simulink model "gap_generation_platoon_alternative"  (R2019a)
settings: Solver=VariableStepAuto  StartTime=0.0  StopTime=50  RelTol=1e-3
libraries: simulink x35, autolibshared x7, powerlib_meascontrol x3
(part 2 of 3)

== system gap_generation_platoon_alternative/p3 ==
  leaderStates : Inport
  virtualLeaderStates : Inport  Port=2
  lcFlag : Inport  Port=3
  activate ACC-v : Inport  Port=4
  ACC : Subsystem
  ACC-v : Subsystem
  AND : Logic  Inputs=3  IconShape=distinctive  AllPortsSameDT=off  OutDataTypeStr=boolean
  Abs : Abs
  Abs1 : Abs  ZeroCross=off
  Bus Creator : BusCreator  Inputs=4
  Bus Selector : BusSelector  OutputSignals=InertFrm.RearAxl.Disp.X,InertFrm.RearAxl.Disp.Y,InertFrm.RearAxl.Vel.Xdot
  Compare To Constant : simulink/Logic and Bit Operations/Compare To Constant  relop=<=  const=0.5  OutDataTypeStr=boolean
  Compare To Constant1 : simulink/Logic and Bit Operations/Compare To Constant  relop=<=  const=0.5  OutDataTypeStr=boolean
  Constant : Constant  Value=0
  Constant1 : Constant  Value=maxAcceleration+1
  Constant2 : Constant  Value=0
  Gain : Gain  Gain=m/2
  Min : MinMax  Inputs=2
  Mux1 : Mux  Inputs=6
  On Delay : powerlib_meascontrol/Logic/On Delay  DelayType=On delay  delay=1  ic=0  Ts=0
      settings: SourceProductName=Simscape Electrical
  Scope : Scope  NumInputPorts=2
  Signal Specification : SignalSpecification  Dimensions=1
  Switch : Switch  Criteria=u2 > Threshold
  Terminator : Terminator
  Transport Delay : TransportDelay
  Triggered Subsystem : Subsystem  TreatAsAtomicUnit=on
  Vehicle Body 3DOF Single Track : autolibshared/Vehicle Body 3DOF Single Track  trackMode=Single (bicycle)  inputMode=External longitudinal forces  frontSteerMode=on  rearSteerMode=off  windMode=off  muMode=off  extFMode=off  extMMode=off  extXo=off  extpsio=off  extxdoto=off  extro=off  extYo=off  extTamb=off  extydoto=off  aMode=2  NF=2  NR=2  m=m  a=lf  b=lr  h=0.35  X_o=x0  xdot_o=vx0  CalphaMode=off  sigmaMode=on  d=0  w=[1.4,1.4]  Cy_f=12e3  Cy_r=11e3  sigma_f=.1  sigma_r=.1  alpha_f_brk=[-.1 .1]  Cy_f_data=[-9e3 9e3]  alpha_r_brk=[-.1 .1]  Cy_r_data=[-9e3 9e3]  Y_o=y0  ydot_o=0  Izz=4000  psi_o=0  r_o=0  Af=2  Cd=.3  Cl=.1  Cpm=.1  beta_w=[0:0.01:0.3]  Cs=[0:0.03:0.9]  Cym=[0:0.01:0.3]  Pabs=101325  Tair=273  g=9.81  mu=1  xdot_tol=.01  Fznom=5000  Fxtire_sat=7e4  Fytire_sat=7e4  longOff=0  latOff=0  vertOff=0  wrapAng=off
      settings: SourceProductName=Powertrain Blockset  SourceProductBaseCode=PW
  states : Outport
  errors : Outport  Port=2
  gap : Outport  Port=3
  virtualErrors : Outport  Port=4
  virtualGap : Outport  Port=5
  gapRequest : Outport  Port=6
  wires:
  Bus Selector/3 -> Bus Creator/3  "<Xdot>"
  Bus Selector/1 -> Bus Creator/1  "<X>"
  Min/1 -> Signal Specification/1  "u"
  ACC/1(u) -> Min/1  "acc"
  Gain/1 -> Vehicle Body 3DOF Single Track/3, Vehicle Body 3DOF Single Track/2
  Constant/1 -> Vehicle Body 3DOF Single Track/1
  Vehicle Body 3DOF Single Track/1 -> Bus Selector/1
  Vehicle Body 3DOF Single Track/4 -> Mux1/3
  Vehicle Body 3DOF Single Track/3 -> Mux1/2
  Vehicle Body 3DOF Single Track/2 -> Mux1/1
  Vehicle Body 3DOF Single Track/5 -> Mux1/4
  Vehicle Body 3DOF Single Track/6 -> Mux1/5
  Vehicle Body 3DOF Single Track/7 -> Mux1/6
  Mux1/1 -> Terminator/1
  ACC/3(gap) -> gap/1
  Bus Creator/1 -> ACC/1(currentStates), ACC-v/1(currentStates), states/1
  leaderStates/1 -> ACC/2(leaderStates)
  virtualLeaderStates/1 -> ACC-v/2(leaderStates)
  ACC/2(errors) -> errors/1
  Switch/1 -> Min/2  "acc-v"
  ACC-v/1(u) -> Switch/1
  ACC-v/2(errors) -> virtualErrors/1
  ACC-v/3(gap) -> virtualGap/1
  Bus Selector/2 -> Bus Creator/2  "<Y>"
  Signal Specification/1 -> Transport Delay/1, Abs1/1, Bus Creator/4, Gain/1
  activate ACC-v/1 -> ACC-v/3(activate), Switch/2
  Constant1/1 -> Switch/3
  AND/1 -> Triggered Subsystem/Trigger
  Compare To Constant1/1 -> Scope/1, AND/1
  On Delay/1 -> AND/3, Triggered Subsystem/1(In1)
  Triggered Subsystem/1(Out1) -> Scope/2
  Compare To Constant/1 -> AND/2
  Transport Delay/1 -> Abs/1
  Abs/1 -> Compare To Constant/1
  Abs1/1 -> Compare To Constant1/1
  lcFlag/1 -> ACC-v/4(lcFlag), gapRequest/1, On Delay/1
  Constant2/1 -> ACC/3(lcFlag)

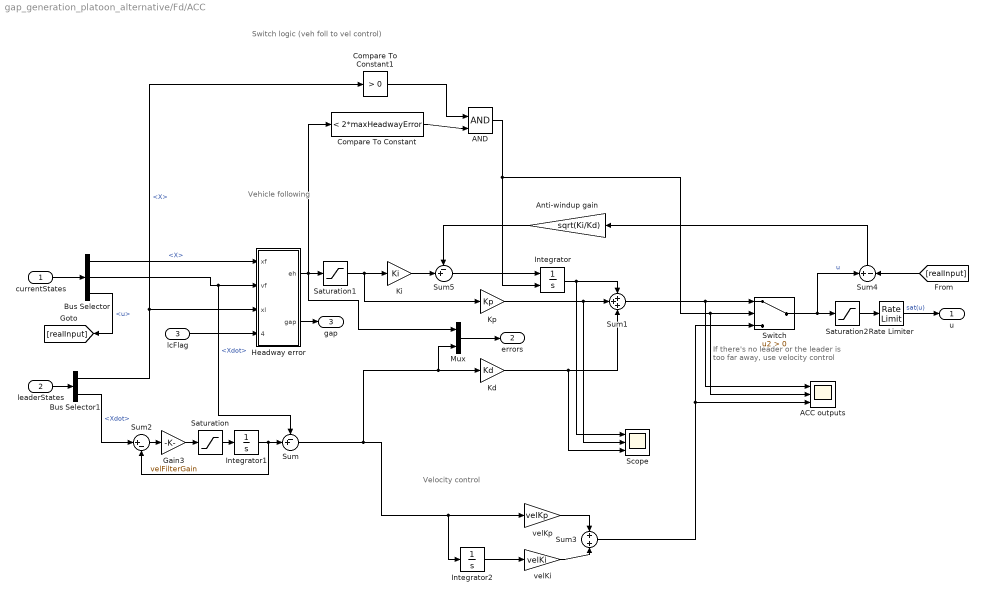
== system gap_generation_platoon_alternative/Fd/ACC ==
  note: Vehicle following
  note: Switch logic (veh foll to vel control)
  note: Velocity control
  note: If there's no leader or the leader
      | is too far away, use velocity control
  currentStates : Inport
  leaderStates : Inport  Port=2
  lcFlag : Inport  Port=3
  ACC outputs : Scope  NumInputPorts=3
  AND : Logic  IconShape=distinctive  AllPortsSameDT=off  OutDataTypeStr=boolean
  Anti-windup gain : Gain  Gain=sqrt(Ki/Kd)
  Bus Selector : BusSelector  OutputSignals=X,Xdot,u
  Bus Selector1 : BusSelector  OutputSignals=X,Xdot
  Compare To Constant : simulink/Logic and Bit Operations/Compare To Constant  relop=<  const=2*maxHeadwayError  OutDataTypeStr=boolean
  Compare To Constant1 : simulink/Logic and Bit Operations/Compare To Constant  relop=>  const=0  OutDataTypeStr=boolean
  Gain3 : Gain  Gain=velFilterGain
  Headway error : Subsystem
  Integrator : Integrator  ExternalReset=either
  Integrator1 : Integrator  InitialCondition=vx0
  Integrator2 : Integrator
  Kd : Gain  Gain=Kd
  Ki : Gain  Gain=Ki
  Kp : Gain  Gain=Kp
  Mux : Mux  Inputs=2
  Rate Limiter : RateLimiter  RisingSlewLimit=maxJerk  FallingSlewLimit=minJerk  SampleTimeMode=inherited
  Saturation : Saturate  UpperLimit=maxAcceleration  LowerLimit=minAcceleration
  Saturation1 : Saturate  UpperLimit=maxHeadwayError  LowerLimit=minHeadwayError
  Saturation2 : Saturate  UpperLimit=maxAcceleration  LowerLimit=minAcceleration
  Scope : Scope  NumInputPorts=3
  Sum : Sum  Inputs=-+|
  Sum1 : Sum  Inputs=+++
  Sum2 : Sum  Inputs=|+-
  Sum3 : Sum
  Sum4 : Sum  Inputs=+-
  Sum5 : Sum  Inputs=-+|
  Switch : Switch  Criteria=u2 > Threshold
  velKi : Gain  Gain=velKi
  velKp : Gain  Gain=velKp
  u : Outport
  errors : Outport  Port=2
  gap : Outport  Port=3
  wires:
  Headway error/1(eh) -> Mux/1, Compare To Constant/1, Saturation1/1
  Bus Selector/2 -> Headway error/2(vf), Sum/1  "<Xdot>"
  Kd/1 -> Scope/3, Sum1/3
  Kp/1 -> Scope/2, Sum1/2
  Gain3/1 -> Saturation/1
  Saturation/1 -> Integrator1/1
  Integrator1/1 -> Sum2/2, Sum/2
  Bus Selector1/2 -> Sum2/1  "<Xdot>"
  Sum2/1 -> Gain3/1
  Saturation1/1 -> Kp/1, Ki/1
  Headway error/2("gap ") -> gap/1
  Integrator2/1 -> velKi/1
  velKi/1 -> Sum3/2
  Switch/1 -> Sum4/1, Saturation2/1  "u"
  Sum1/1 -> Switch/1, ACC outputs/1
  Sum3/1 -> ACC outputs/3, Switch/3
  Sum/1 -> Mux/2, Kd/1, velKp/1, Integrator2/1
  Mux/1 -> errors/1
  Saturation2/1 -> Rate Limiter/1
  Sum4/1 -> Anti-windup gain/1
  Sum5/1 -> Integrator/1
  Rate Limiter/1 -> u/1  "sat(u)"
  velKp/1 -> Sum3/1
  Ki/1 -> Sum5/2
  Integrator/1 -> Sum1/1, Scope/1
  Anti-windup gain/1 -> Sum5/1
  AND/1 -> Integrator/2, Switch/2, ACC outputs/2
  Compare To Constant/1 -> AND/2
  Compare To Constant1/1 -> AND/1
  lcFlag/1 -> Headway error/4(lcFlag)
  currentStates/1 -> Bus Selector/1
  Bus Selector/1 -> Headway error/1(xf)  "<X>"
  leaderStates/1 -> Bus Selector1/1
  Bus Selector1/1 -> Compare To Constant1/1, Headway error/3(xl)  "<X>"
  Bus Selector/3 -> [realInput]  "<u>"
  [realInput] -> Sum4/2

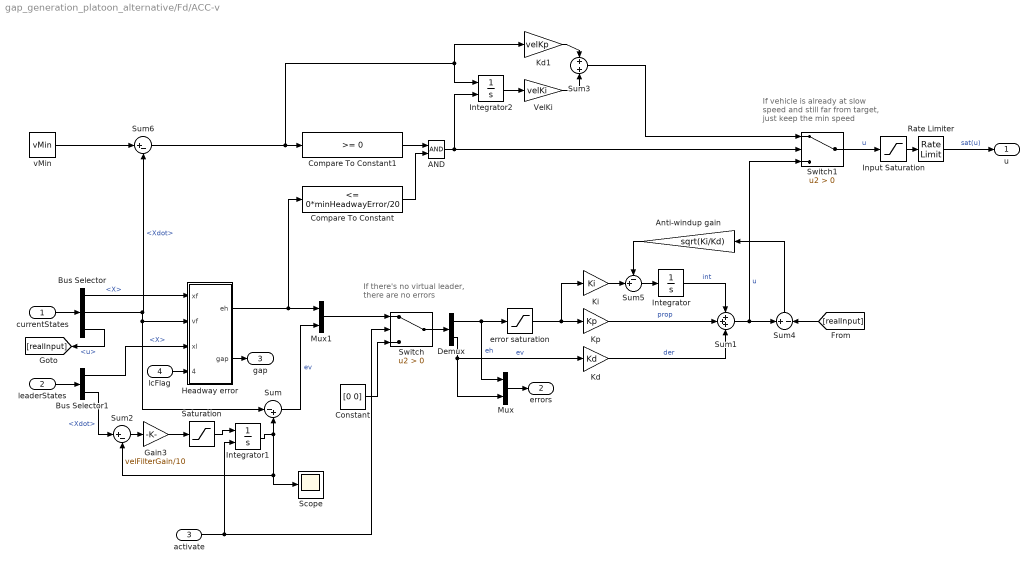
== system gap_generation_platoon_alternative/Fd/ACC-v ==
  note: If vehicle is already at slow
      | speed and still far from target,
      | just keep the min speed
  note: If there's no virtual leader,
      | there are no errors
  currentStates : Inport
  leaderStates : Inport  Port=2
  activate : Inport  Port=3
  lcFlag : Inport  Port=4
  AND : Logic  IconShape=distinctive  AllPortsSameDT=off  OutDataTypeStr=boolean
  Anti-windup gain : Gain  Gain=sqrt(Ki/Kd)
  Bus Selector : BusSelector  OutputSignals=X,Xdot,u
  Bus Selector1 : BusSelector  OutputSignals=X,Xdot
  Compare To Constant : simulink/Logic and Bit Operations/Compare To Constant  relop=<=  const=0*minHeadwayError/20  OutDataTypeStr=boolean
  Compare To Constant1 : simulink/Logic and Bit Operations/Compare To Constant  relop=>=  const=0  OutDataTypeStr=boolean
  Constant : Constant  Value=[0 0]
  Demux : Demux  Outputs=2
  Gain3 : Gain  Gain=velFilterGain/10
  Headway error : Subsystem
  Input Saturation : Saturate  UpperLimit=maxAcceleration/2  LowerLimit=minAcceleration/4
  Integrator : Integrator
  Integrator1 : Integrator  ExternalReset=rising  InitialCondition=vx0
  Integrator2 : Integrator  ExternalReset=rising
  Kd : Gain  Gain=Kd
  Kd1 : Gain  Gain=velKp
  Ki : Gain  Gain=Ki
  Kp : Gain  Gain=Kp
  Mux : Mux  Inputs=2
  Mux1 : Mux  Inputs=2
  Rate Limiter : RateLimiter  RisingSlewLimit=maxJerk/2  FallingSlewLimit=minJerk/3  SampleTimeMode=inherited
  Saturation : Saturate  UpperLimit=maxAcceleration  LowerLimit=minAcceleration
  Scope : Scope
  Sum : Sum  Inputs=|-+
  Sum1 : Sum  Inputs=+++
  Sum2 : Sum  Inputs=|+-
  Sum3 : Sum
  Sum4 : Sum  Inputs=+-
  Sum5 : Sum  Inputs=-+|
  Sum6 : Sum  Inputs=|+-
  Switch : Switch  Criteria=u2 > Threshold
  Switch1 : Switch  Criteria=u2 > Threshold
  VelKi : Gain  Gain=velKi
  error saturation : Saturate  UpperLimit=maxHeadwayError  LowerLimit=minHeadwayError/10
  vMin : Constant  Value=vMin
  u : Outport
  errors : Outport  Port=2
  gap : Outport  Port=3
  wires:
  Headway error/1(eh) -> Compare To Constant/1, Mux1/1
  Kd/1 -> Sum1/3  "der"
  Kp/1 -> Sum1/2  "prop"
  Gain3/1 -> Saturation/1
  Saturation/1 -> Integrator1/1
  Integrator1/1 -> Scope/1, Sum2/2, Sum/2
  Bus Selector1/2 -> Sum2/1  "<Xdot>"
  Sum2/1 -> Gain3/1
  Demux/1 -> Mux/1, error saturation/1  "eh"
  Headway error/2("gap ") -> gap/1
  Sum1/1 -> Switch1/3, Sum4/1  "u"
  Sum/1 -> Mux1/2  "ev"
  Mux/1 -> errors/1
  Input Saturation/1 -> Rate Limiter/1
  Integrator/1 -> Sum1/1  "int"
  Sum4/1 -> Anti-windup gain/1
  Ki/1 -> Sum5/2
  Anti-windup gain/1 -> Sum5/1
  Demux/2 -> Kd/1, Mux/2  "ev"
  Switch/1 -> Demux/1
  Mux1/1 -> Switch/1
  activate/1 -> Integrator1/2, Switch/2
  Constant/1 -> Switch/3
  Rate Limiter/1 -> u/1  "sat(u)"
  Compare To Constant1/1 -> AND/1
  Compare To Constant/1 -> AND/2
  Sum6/1 -> Integrator2/1, Kd1/1, Compare To Constant1/1
  Sum3/1 -> Switch1/1
  Integrator2/1 -> VelKi/1
  Kd1/1 -> Sum3/1
  VelKi/1 -> Sum3/2
  vMin/1 -> Sum6/1
  Switch1/1 -> Input Saturation/1  "u"
  error saturation/1 -> Kp/1, Ki/1
  Sum5/1 -> Integrator/1
  AND/1 -> Switch1/2, Integrator2/2
  [realInput] -> Sum4/2
  currentStates/1 -> Bus Selector/1
  Bus Selector/1 -> Headway error/1(xf)  "<X>"
  Bus Selector/2 -> Sum6/2, Headway error/2(vf), Sum/1  "<Xdot>"
  leaderStates/1 -> Bus Selector1/1
  Bus Selector1/1 -> Headway error/3(xl)  "<X>"
  Bus Selector/3 -> [realInput]  "<u>"
  lcFlag/1 -> Headway error/4(lcFlag)

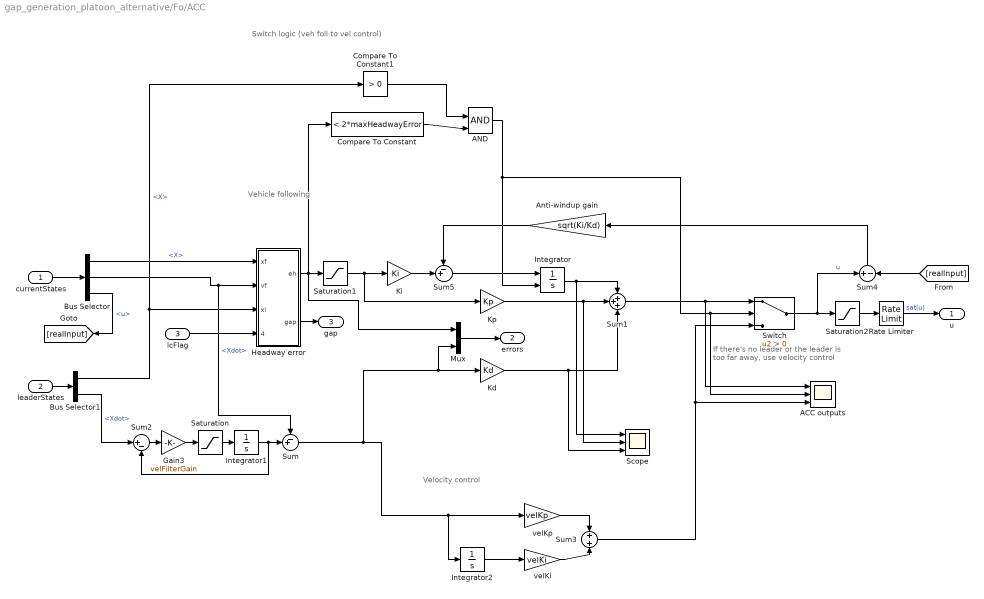
== system gap_generation_platoon_alternative/Fo/ACC ==
  note: Vehicle following
  note: Switch logic (veh foll to vel control)
  note: Velocity control
  note: If there's no leader or the leader
      | is too far away, use velocity control
  currentStates : Inport
  leaderStates : Inport  Port=2
  lcFlag : Inport  Port=3
  ACC outputs : Scope  NumInputPorts=3
  AND : Logic  IconShape=distinctive  AllPortsSameDT=off  OutDataTypeStr=boolean
  Anti-windup gain : Gain  Gain=sqrt(Ki/Kd)
  Bus Selector : BusSelector  OutputSignals=X,Xdot,u
  Bus Selector1 : BusSelector  OutputSignals=X,Xdot
  Compare To Constant : simulink/Logic and Bit Operations/Compare To Constant  relop=<  const=2*maxHeadwayError  OutDataTypeStr=boolean
  Compare To Constant1 : simulink/Logic and Bit Operations/Compare To Constant  relop=>  const=0  OutDataTypeStr=boolean
  Gain3 : Gain  Gain=velFilterGain
  Headway error : Subsystem
  Integrator : Integrator  ExternalReset=either
  Integrator1 : Integrator  InitialCondition=vx0
  Integrator2 : Integrator
  Kd : Gain  Gain=Kd
  Ki : Gain  Gain=Ki
  Kp : Gain  Gain=Kp
  Mux : Mux  Inputs=2
  Rate Limiter : RateLimiter  RisingSlewLimit=maxJerk  FallingSlewLimit=minJerk  SampleTimeMode=inherited
  Saturation : Saturate  UpperLimit=maxAcceleration  LowerLimit=minAcceleration
  Saturation1 : Saturate  UpperLimit=maxHeadwayError  LowerLimit=minHeadwayError
  Saturation2 : Saturate  UpperLimit=maxAcceleration  LowerLimit=minAcceleration
  Scope : Scope  NumInputPorts=3
  Sum : Sum  Inputs=-+|
  Sum1 : Sum  Inputs=+++
  Sum2 : Sum  Inputs=|+-
  Sum3 : Sum
  Sum4 : Sum  Inputs=+-
  Sum5 : Sum  Inputs=-+|
  Switch : Switch  Criteria=u2 > Threshold
  velKi : Gain  Gain=velKi
  velKp : Gain  Gain=velKp
  u : Outport
  errors : Outport  Port=2
  gap : Outport  Port=3
  wires:
  Headway error/1(eh) -> Mux/1, Compare To Constant/1, Saturation1/1
  Bus Selector/2 -> Headway error/2(vf), Sum/1  "<Xdot>"
  Kd/1 -> Scope/3, Sum1/3
  Kp/1 -> Scope/2, Sum1/2
  Gain3/1 -> Saturation/1
  Saturation/1 -> Integrator1/1
  Integrator1/1 -> Sum2/2, Sum/2
  Bus Selector1/2 -> Sum2/1  "<Xdot>"
  Sum2/1 -> Gain3/1
  Saturation1/1 -> Kp/1, Ki/1
  Headway error/2("gap ") -> gap/1
  Integrator2/1 -> velKi/1
  velKi/1 -> Sum3/2
  Switch/1 -> Sum4/1, Saturation2/1  "u"
  Sum1/1 -> Switch/1, ACC outputs/1
  Sum3/1 -> ACC outputs/3, Switch/3
  Sum/1 -> Mux/2, Kd/1, velKp/1, Integrator2/1
  Mux/1 -> errors/1
  Saturation2/1 -> Rate Limiter/1
  Sum4/1 -> Anti-windup gain/1
  Sum5/1 -> Integrator/1
  Rate Limiter/1 -> u/1  "sat(u)"
  velKp/1 -> Sum3/1
  Ki/1 -> Sum5/2
  Integrator/1 -> Sum1/1, Scope/1
  Anti-windup gain/1 -> Sum5/1
  AND/1 -> Integrator/2, Switch/2, ACC outputs/2
  Compare To Constant/1 -> AND/2
  Compare To Constant1/1 -> AND/1
  lcFlag/1 -> Headway error/4(lcFlag)
  currentStates/1 -> Bus Selector/1
  Bus Selector/1 -> Headway error/1(xf)  "<X>"
  leaderStates/1 -> Bus Selector1/1
  Bus Selector1/1 -> Compare To Constant1/1, Headway error/3(xl)  "<X>"
  Bus Selector/3 -> [realInput]  "<u>"
  [realInput] -> Sum4/2

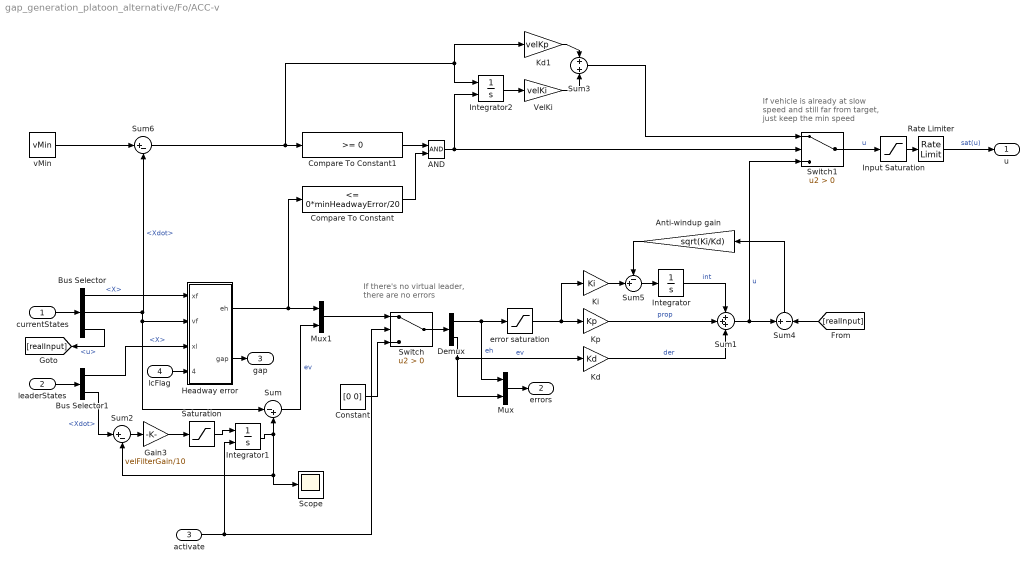
== system gap_generation_platoon_alternative/Fo/ACC-v ==
  note: If vehicle is already at slow
      | speed and still far from target,
      | just keep the min speed
  note: If there's no virtual leader,
      | there are no errors
  currentStates : Inport
  leaderStates : Inport  Port=2
  activate : Inport  Port=3
  lcFlag : Inport  Port=4
  AND : Logic  IconShape=distinctive  AllPortsSameDT=off  OutDataTypeStr=boolean
  Anti-windup gain : Gain  Gain=sqrt(Ki/Kd)
  Bus Selector : BusSelector  OutputSignals=X,Xdot,u
  Bus Selector1 : BusSelector  OutputSignals=X,Xdot
  Compare To Constant : simulink/Logic and Bit Operations/Compare To Constant  relop=<=  const=0*minHeadwayError/20  OutDataTypeStr=boolean
  Compare To Constant1 : simulink/Logic and Bit Operations/Compare To Constant  relop=>=  const=0  OutDataTypeStr=boolean
  Constant : Constant  Value=[0 0]
  Demux : Demux  Outputs=2
  Gain3 : Gain  Gain=velFilterGain/10
  Headway error : Subsystem
  Input Saturation : Saturate  UpperLimit=maxAcceleration/2  LowerLimit=minAcceleration/4
  Integrator : Integrator
  Integrator1 : Integrator  ExternalReset=rising  InitialCondition=vx0
  Integrator2 : Integrator  ExternalReset=rising
  Kd : Gain  Gain=Kd
  Kd1 : Gain  Gain=velKp
  Ki : Gain  Gain=Ki
  Kp : Gain  Gain=Kp
  Mux : Mux  Inputs=2
  Mux1 : Mux  Inputs=2
  Rate Limiter : RateLimiter  RisingSlewLimit=maxJerk/2  FallingSlewLimit=minJerk/3  SampleTimeMode=inherited
  Saturation : Saturate  UpperLimit=maxAcceleration  LowerLimit=minAcceleration
  Scope : Scope
  Sum : Sum  Inputs=|-+
  Sum1 : Sum  Inputs=+++
  Sum2 : Sum  Inputs=|+-
  Sum3 : Sum
  Sum4 : Sum  Inputs=+-
  Sum5 : Sum  Inputs=-+|
  Sum6 : Sum  Inputs=|+-
  Switch : Switch  Criteria=u2 > Threshold
  Switch1 : Switch  Criteria=u2 > Threshold
  VelKi : Gain  Gain=velKi
  error saturation : Saturate  UpperLimit=maxHeadwayError  LowerLimit=minHeadwayError/10
  vMin : Constant  Value=vMin
  u : Outport
  errors : Outport  Port=2
  gap : Outport  Port=3
  wires:
  Headway error/1(eh) -> Compare To Constant/1, Mux1/1
  Kd/1 -> Sum1/3  "der"
  Kp/1 -> Sum1/2  "prop"
  Gain3/1 -> Saturation/1
  Saturation/1 -> Integrator1/1
  Integrator1/1 -> Scope/1, Sum2/2, Sum/2
  Bus Selector1/2 -> Sum2/1  "<Xdot>"
  Sum2/1 -> Gain3/1
  Demux/1 -> Mux/1, error saturation/1  "eh"
  Headway error/2("gap ") -> gap/1
  Sum1/1 -> Switch1/3, Sum4/1  "u"
  Sum/1 -> Mux1/2  "ev"
  Mux/1 -> errors/1
  Input Saturation/1 -> Rate Limiter/1
  Integrator/1 -> Sum1/1  "int"
  Sum4/1 -> Anti-windup gain/1
  Ki/1 -> Sum5/2
  Anti-windup gain/1 -> Sum5/1
  Demux/2 -> Kd/1, Mux/2  "ev"
  Switch/1 -> Demux/1
  Mux1/1 -> Switch/1
  activate/1 -> Integrator1/2, Switch/2
  Constant/1 -> Switch/3
  Rate Limiter/1 -> u/1  "sat(u)"
  Compare To Constant1/1 -> AND/1
  Compare To Constant/1 -> AND/2
  Sum6/1 -> Integrator2/1, Kd1/1, Compare To Constant1/1
  Sum3/1 -> Switch1/1
  Integrator2/1 -> VelKi/1
  Kd1/1 -> Sum3/1
  VelKi/1 -> Sum3/2
  vMin/1 -> Sum6/1
  Switch1/1 -> Input Saturation/1  "u"
  error saturation/1 -> Kp/1, Ki/1
  Sum5/1 -> Integrator/1
  AND/1 -> Switch1/2, Integrator2/2
  [realInput] -> Sum4/2
  currentStates/1 -> Bus Selector/1
  Bus Selector/1 -> Headway error/1(xf)  "<X>"
  Bus Selector/2 -> Sum6/2, Headway error/2(vf), Sum/1  "<Xdot>"
  leaderStates/1 -> Bus Selector1/1
  Bus Selector1/1 -> Headway error/3(xl)  "<X>"
  Bus Selector/3 -> [realInput]  "<u>"
  lcFlag/1 -> Headway error/4(lcFlag)

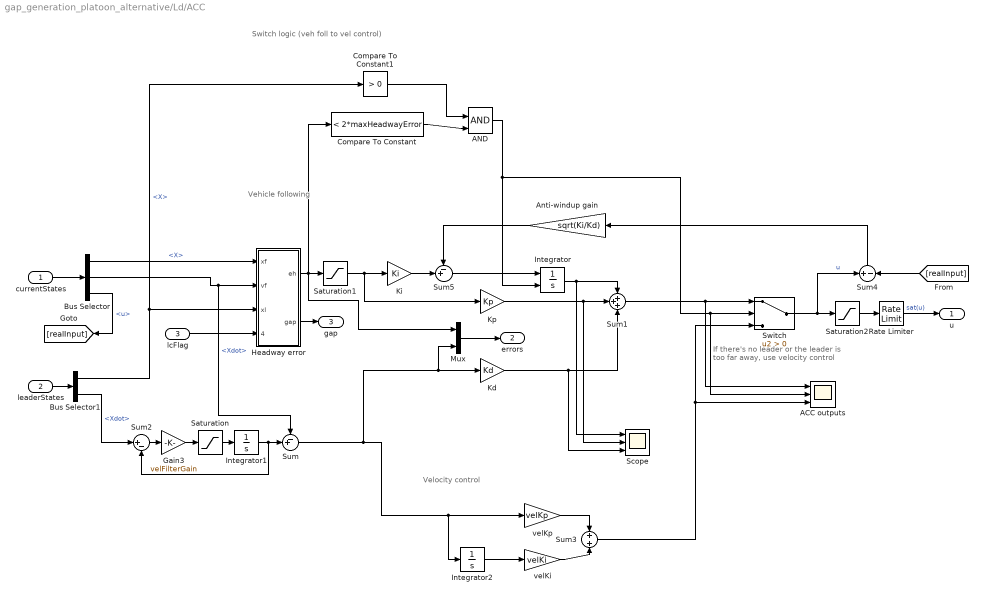
== system gap_generation_platoon_alternative/Ld/ACC ==
  note: Vehicle following
  note: Switch logic (veh foll to vel control)
  note: Velocity control
  note: If there's no leader or the leader
      | is too far away, use velocity control
  currentStates : Inport
  leaderStates : Inport  Port=2
  lcFlag : Inport  Port=3
  ACC outputs : Scope  NumInputPorts=3
  AND : Logic  IconShape=distinctive  AllPortsSameDT=off  OutDataTypeStr=boolean
  Anti-windup gain : Gain  Gain=sqrt(Ki/Kd)
  Bus Selector : BusSelector  OutputSignals=X,Xdot,u
  Bus Selector1 : BusSelector  OutputSignals=X,Xdot
  Compare To Constant : simulink/Logic and Bit Operations/Compare To Constant  relop=<  const=2*maxHeadwayError  OutDataTypeStr=boolean
  Compare To Constant1 : simulink/Logic and Bit Operations/Compare To Constant  relop=>  const=0  OutDataTypeStr=boolean
  Gain3 : Gain  Gain=velFilterGain
  Headway error : Subsystem
  Integrator : Integrator  ExternalReset=either
  Integrator1 : Integrator  InitialCondition=vx0
  Integrator2 : Integrator
  Kd : Gain  Gain=Kd
  Ki : Gain  Gain=Ki
  Kp : Gain  Gain=Kp
  Mux : Mux  Inputs=2
  Rate Limiter : RateLimiter  RisingSlewLimit=maxJerk  FallingSlewLimit=minJerk  SampleTimeMode=inherited
  Saturation : Saturate  UpperLimit=maxAcceleration  LowerLimit=minAcceleration
  Saturation1 : Saturate  UpperLimit=maxHeadwayError  LowerLimit=minHeadwayError
  Saturation2 : Saturate  UpperLimit=maxAcceleration  LowerLimit=minAcceleration
  Scope : Scope  NumInputPorts=3
  Sum : Sum  Inputs=-+|
  Sum1 : Sum  Inputs=+++
  Sum2 : Sum  Inputs=|+-
  Sum3 : Sum
  Sum4 : Sum  Inputs=+-
  Sum5 : Sum  Inputs=-+|
  Switch : Switch  Criteria=u2 > Threshold
  velKi : Gain  Gain=velKi
  velKp : Gain  Gain=velKp
  u : Outport
  errors : Outport  Port=2
  gap : Outport  Port=3
  wires:
  Headway error/1(eh) -> Mux/1, Compare To Constant/1, Saturation1/1
  Bus Selector/2 -> Headway error/2(vf), Sum/1  "<Xdot>"
  Kd/1 -> Scope/3, Sum1/3
  Kp/1 -> Scope/2, Sum1/2
  Gain3/1 -> Saturation/1
  Saturation/1 -> Integrator1/1
  Integrator1/1 -> Sum2/2, Sum/2
  Bus Selector1/2 -> Sum2/1  "<Xdot>"
  Sum2/1 -> Gain3/1
  Saturation1/1 -> Kp/1, Ki/1
  Headway error/2("gap ") -> gap/1
  Integrator2/1 -> velKi/1
  velKi/1 -> Sum3/2
  Switch/1 -> Sum4/1, Saturation2/1  "u"
  Sum1/1 -> Switch/1, ACC outputs/1
  Sum3/1 -> ACC outputs/3, Switch/3
  Sum/1 -> Mux/2, Kd/1, velKp/1, Integrator2/1
  Mux/1 -> errors/1
  Saturation2/1 -> Rate Limiter/1
  Sum4/1 -> Anti-windup gain/1
  Sum5/1 -> Integrator/1
  Rate Limiter/1 -> u/1  "sat(u)"
  velKp/1 -> Sum3/1
  Ki/1 -> Sum5/2
  Integrator/1 -> Sum1/1, Scope/1
  Anti-windup gain/1 -> Sum5/1
  AND/1 -> Integrator/2, Switch/2, ACC outputs/2
  Compare To Constant/1 -> AND/2
  Compare To Constant1/1 -> AND/1
  lcFlag/1 -> Headway error/4(lcFlag)
  currentStates/1 -> Bus Selector/1
  Bus Selector/1 -> Headway error/1(xf)  "<X>"
  leaderStates/1 -> Bus Selector1/1
  Bus Selector1/1 -> Compare To Constant1/1, Headway error/3(xl)  "<X>"
  Bus Selector/3 -> [realInput]  "<u>"
  [realInput] -> Sum4/2

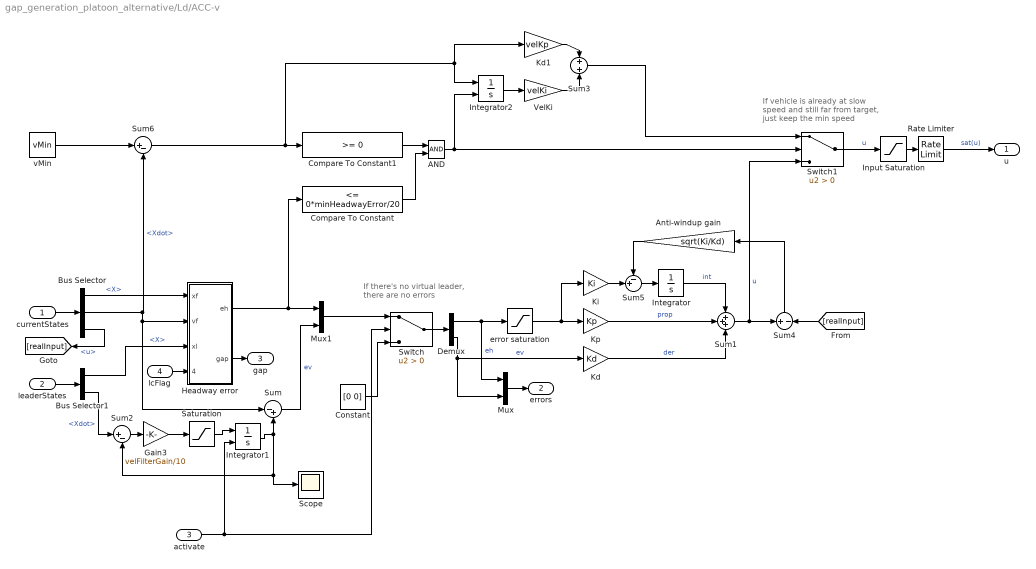
== system gap_generation_platoon_alternative/Ld/ACC-v ==
  note: If vehicle is already at slow
      | speed and still far from target,
      | just keep the min speed
  note: If there's no virtual leader,
      | there are no errors
  currentStates : Inport
  leaderStates : Inport  Port=2
  activate : Inport  Port=3
  lcFlag : Inport  Port=4
  AND : Logic  IconShape=distinctive  AllPortsSameDT=off  OutDataTypeStr=boolean
  Anti-windup gain : Gain  Gain=sqrt(Ki/Kd)
  Bus Selector : BusSelector  OutputSignals=X,Xdot,u
  Bus Selector1 : BusSelector  OutputSignals=X,Xdot
  Compare To Constant : simulink/Logic and Bit Operations/Compare To Constant  relop=<=  const=0*minHeadwayError/20  OutDataTypeStr=boolean
  Compare To Constant1 : simulink/Logic and Bit Operations/Compare To Constant  relop=>=  const=0  OutDataTypeStr=boolean
  Constant : Constant  Value=[0 0]
  Demux : Demux  Outputs=2
  Gain3 : Gain  Gain=velFilterGain/10
  Headway error : Subsystem
  Input Saturation : Saturate  UpperLimit=maxAcceleration/2  LowerLimit=minAcceleration/4
  Integrator : Integrator
  Integrator1 : Integrator  ExternalReset=rising  InitialCondition=vx0
  Integrator2 : Integrator  ExternalReset=rising
  Kd : Gain  Gain=Kd
  Kd1 : Gain  Gain=velKp
  Ki : Gain  Gain=Ki
  Kp : Gain  Gain=Kp
  Mux : Mux  Inputs=2
  Mux1 : Mux  Inputs=2
  Rate Limiter : RateLimiter  RisingSlewLimit=maxJerk/2  FallingSlewLimit=minJerk/3  SampleTimeMode=inherited
  Saturation : Saturate  UpperLimit=maxAcceleration  LowerLimit=minAcceleration
  Scope : Scope
  Sum : Sum  Inputs=|-+
  Sum1 : Sum  Inputs=+++
  Sum2 : Sum  Inputs=|+-
  Sum3 : Sum
  Sum4 : Sum  Inputs=+-
  Sum5 : Sum  Inputs=-+|
  Sum6 : Sum  Inputs=|+-
  Switch : Switch  Criteria=u2 > Threshold
  Switch1 : Switch  Criteria=u2 > Threshold
  VelKi : Gain  Gain=velKi
  error saturation : Saturate  UpperLimit=maxHeadwayError  LowerLimit=minHeadwayError/10
  vMin : Constant  Value=vMin
  u : Outport
  errors : Outport  Port=2
  gap : Outport  Port=3
  wires:
  Headway error/1(eh) -> Compare To Constant/1, Mux1/1
  Kd/1 -> Sum1/3  "der"
  Kp/1 -> Sum1/2  "prop"
  Gain3/1 -> Saturation/1
  Saturation/1 -> Integrator1/1
  Integrator1/1 -> Scope/1, Sum2/2, Sum/2
  Bus Selector1/2 -> Sum2/1  "<Xdot>"
  Sum2/1 -> Gain3/1
  Demux/1 -> Mux/1, error saturation/1  "eh"
  Headway error/2("gap ") -> gap/1
  Sum1/1 -> Switch1/3, Sum4/1  "u"
  Sum/1 -> Mux1/2  "ev"
  Mux/1 -> errors/1
  Input Saturation/1 -> Rate Limiter/1
  Integrator/1 -> Sum1/1  "int"
  Sum4/1 -> Anti-windup gain/1
  Ki/1 -> Sum5/2
  Anti-windup gain/1 -> Sum5/1
  Demux/2 -> Kd/1, Mux/2  "ev"
  Switch/1 -> Demux/1
  Mux1/1 -> Switch/1
  activate/1 -> Integrator1/2, Switch/2
  Constant/1 -> Switch/3
  Rate Limiter/1 -> u/1  "sat(u)"
  Compare To Constant1/1 -> AND/1
  Compare To Constant/1 -> AND/2
  Sum6/1 -> Integrator2/1, Kd1/1, Compare To Constant1/1
  Sum3/1 -> Switch1/1
  Integrator2/1 -> VelKi/1
  Kd1/1 -> Sum3/1
  VelKi/1 -> Sum3/2
  vMin/1 -> Sum6/1
  Switch1/1 -> Input Saturation/1  "u"
  error saturation/1 -> Kp/1, Ki/1
  Sum5/1 -> Integrator/1
  AND/1 -> Switch1/2, Integrator2/2
  [realInput] -> Sum4/2
  currentStates/1 -> Bus Selector/1
  Bus Selector/1 -> Headway error/1(xf)  "<X>"
  Bus Selector/2 -> Sum6/2, Headway error/2(vf), Sum/1  "<Xdot>"
  leaderStates/1 -> Bus Selector1/1
  Bus Selector1/1 -> Headway error/3(xl)  "<X>"
  Bus Selector/3 -> [realInput]  "<u>"
  lcFlag/1 -> Headway error/4(lcFlag)

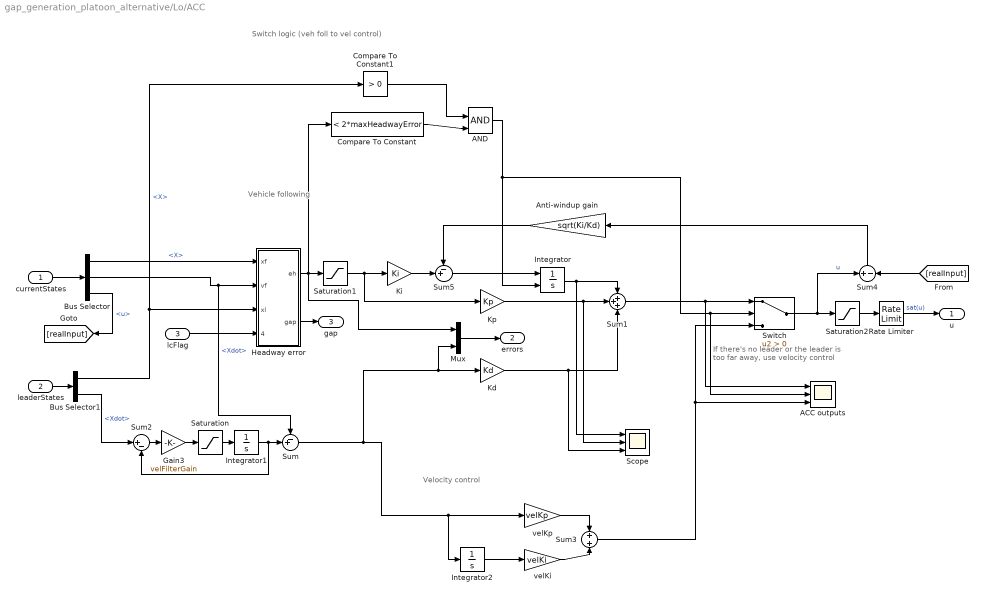
== system gap_generation_platoon_alternative/Lo/ACC ==
  note: Vehicle following
  note: Switch logic (veh foll to vel control)
  note: Velocity control
  note: If there's no leader or the leader
      | is too far away, use velocity control
  currentStates : Inport
  leaderStates : Inport  Port=2
  lcFlag : Inport  Port=3
  ACC outputs : Scope  NumInputPorts=3
  AND : Logic  IconShape=distinctive  AllPortsSameDT=off  OutDataTypeStr=boolean
  Anti-windup gain : Gain  Gain=sqrt(Ki/Kd)
  Bus Selector : BusSelector  OutputSignals=X,Xdot,u
  Bus Selector1 : BusSelector  OutputSignals=X,Xdot
  Compare To Constant : simulink/Logic and Bit Operations/Compare To Constant  relop=<  const=2*maxHeadwayError  OutDataTypeStr=boolean
  Compare To Constant1 : simulink/Logic and Bit Operations/Compare To Constant  relop=>  const=0  OutDataTypeStr=boolean
  Gain3 : Gain  Gain=velFilterGain
  Headway error : Subsystem
  Integrator : Integrator  ExternalReset=either
  Integrator1 : Integrator  InitialCondition=vx0
  Integrator2 : Integrator
  Kd : Gain  Gain=Kd
  Ki : Gain  Gain=Ki
  Kp : Gain  Gain=Kp
  Mux : Mux  Inputs=2
  Rate Limiter : RateLimiter  RisingSlewLimit=maxJerk  FallingSlewLimit=minJerk  SampleTimeMode=inherited
  Saturation : Saturate  UpperLimit=maxAcceleration  LowerLimit=minAcceleration
  Saturation1 : Saturate  UpperLimit=maxHeadwayError  LowerLimit=minHeadwayError
  Saturation2 : Saturate  UpperLimit=maxAcceleration  LowerLimit=minAcceleration
  Scope : Scope  NumInputPorts=3
  Sum : Sum  Inputs=-+|
  Sum1 : Sum  Inputs=+++
  Sum2 : Sum  Inputs=|+-
  Sum3 : Sum
  Sum4 : Sum  Inputs=+-
  Sum5 : Sum  Inputs=-+|
  Switch : Switch  Criteria=u2 > Threshold
  velKi : Gain  Gain=velKi
  velKp : Gain  Gain=velKp
  u : Outport
  errors : Outport  Port=2
  gap : Outport  Port=3
  wires:
  Headway error/1(eh) -> Mux/1, Compare To Constant/1, Saturation1/1
  Bus Selector/2 -> Headway error/2(vf), Sum/1  "<Xdot>"
  Kd/1 -> Scope/3, Sum1/3
  Kp/1 -> Scope/2, Sum1/2
  Gain3/1 -> Saturation/1
  Saturation/1 -> Integrator1/1
  Integrator1/1 -> Sum2/2, Sum/2
  Bus Selector1/2 -> Sum2/1  "<Xdot>"
  Sum2/1 -> Gain3/1
  Saturation1/1 -> Kp/1, Ki/1
  Headway error/2("gap ") -> gap/1
  Integrator2/1 -> velKi/1
  velKi/1 -> Sum3/2
  Switch/1 -> Sum4/1, Saturation2/1  "u"
  Sum1/1 -> Switch/1, ACC outputs/1
  Sum3/1 -> ACC outputs/3, Switch/3
  Sum/1 -> Mux/2, Kd/1, velKp/1, Integrator2/1
  Mux/1 -> errors/1
  Saturation2/1 -> Rate Limiter/1
  Sum4/1 -> Anti-windup gain/1
  Sum5/1 -> Integrator/1
  Rate Limiter/1 -> u/1  "sat(u)"
  velKp/1 -> Sum3/1
  Ki/1 -> Sum5/2
  Integrator/1 -> Sum1/1, Scope/1
  Anti-windup gain/1 -> Sum5/1
  AND/1 -> Integrator/2, Switch/2, ACC outputs/2
  Compare To Constant/1 -> AND/2
  Compare To Constant1/1 -> AND/1
  lcFlag/1 -> Headway error/4(lcFlag)
  currentStates/1 -> Bus Selector/1
  Bus Selector/1 -> Headway error/1(xf)  "<X>"
  leaderStates/1 -> Bus Selector1/1
  Bus Selector1/1 -> Compare To Constant1/1, Headway error/3(xl)  "<X>"
  Bus Selector/3 -> [realInput]  "<u>"
  [realInput] -> Sum4/2

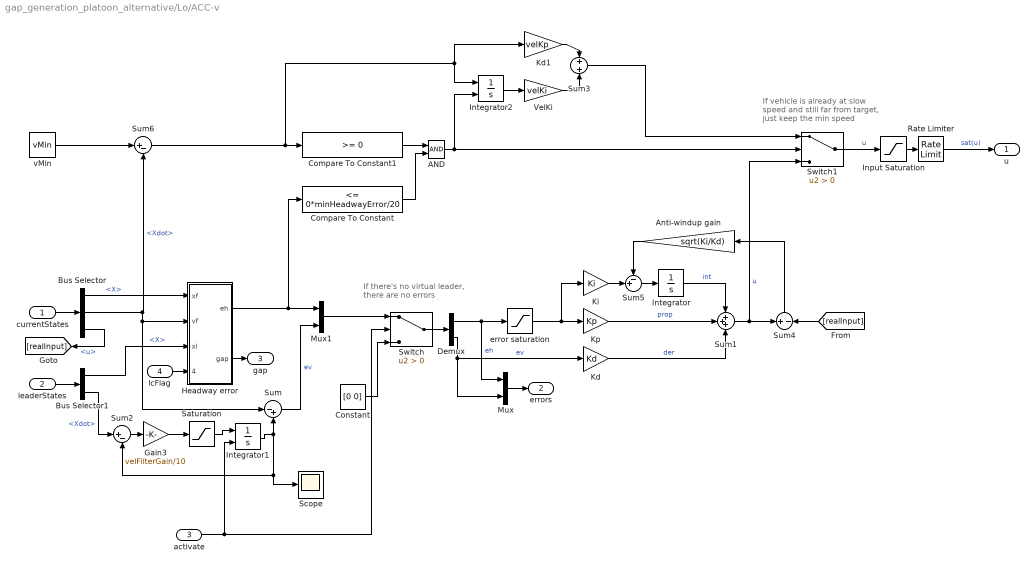
== system gap_generation_platoon_alternative/Lo/ACC-v ==
  note: If vehicle is already at slow
      | speed and still far from target,
      | just keep the min speed
  note: If there's no virtual leader,
      | there are no errors
  currentStates : Inport
  leaderStates : Inport  Port=2
  activate : Inport  Port=3
  lcFlag : Inport  Port=4
  AND : Logic  IconShape=distinctive  AllPortsSameDT=off  OutDataTypeStr=boolean
  Anti-windup gain : Gain  Gain=sqrt(Ki/Kd)
  Bus Selector : BusSelector  OutputSignals=X,Xdot,u
  Bus Selector1 : BusSelector  OutputSignals=X,Xdot
  Compare To Constant : simulink/Logic and Bit Operations/Compare To Constant  relop=<=  const=0*minHeadwayError/20  OutDataTypeStr=boolean
  Compare To Constant1 : simulink/Logic and Bit Operations/Compare To Constant  relop=>=  const=0  OutDataTypeStr=boolean
  Constant : Constant  Value=[0 0]
  Demux : Demux  Outputs=2
  Gain3 : Gain  Gain=velFilterGain/10
  Headway error : Subsystem
  Input Saturation : Saturate  UpperLimit=maxAcceleration/2  LowerLimit=minAcceleration/4
  Integrator : Integrator
  Integrator1 : Integrator  ExternalReset=rising  InitialCondition=vx0
  Integrator2 : Integrator  ExternalReset=rising
  Kd : Gain  Gain=Kd
  Kd1 : Gain  Gain=velKp
  Ki : Gain  Gain=Ki
  Kp : Gain  Gain=Kp
  Mux : Mux  Inputs=2
  Mux1 : Mux  Inputs=2
  Rate Limiter : RateLimiter  RisingSlewLimit=maxJerk/2  FallingSlewLimit=minJerk/3  SampleTimeMode=inherited
  Saturation : Saturate  UpperLimit=maxAcceleration  LowerLimit=minAcceleration
  Scope : Scope
  Sum : Sum  Inputs=|-+
  Sum1 : Sum  Inputs=+++
  Sum2 : Sum  Inputs=|+-
  Sum3 : Sum
  Sum4 : Sum  Inputs=+-
  Sum5 : Sum  Inputs=-+|
  Sum6 : Sum  Inputs=|+-
  Switch : Switch  Criteria=u2 > Threshold
  Switch1 : Switch  Criteria=u2 > Threshold
  VelKi : Gain  Gain=velKi
  error saturation : Saturate  UpperLimit=maxHeadwayError  LowerLimit=minHeadwayError/10
  vMin : Constant  Value=vMin
  u : Outport
  errors : Outport  Port=2
  gap : Outport  Port=3
  wires:
  Headway error/1(eh) -> Compare To Constant/1, Mux1/1
  Kd/1 -> Sum1/3  "der"
  Kp/1 -> Sum1/2  "prop"
  Gain3/1 -> Saturation/1
  Saturation/1 -> Integrator1/1
  Integrator1/1 -> Scope/1, Sum2/2, Sum/2
  Bus Selector1/2 -> Sum2/1  "<Xdot>"
  Sum2/1 -> Gain3/1
  Demux/1 -> Mux/1, error saturation/1  "eh"
  Headway error/2("gap ") -> gap/1
  Sum1/1 -> Switch1/3, Sum4/1  "u"
  Sum/1 -> Mux1/2  "ev"
  Mux/1 -> errors/1
  Input Saturation/1 -> Rate Limiter/1
  Integrator/1 -> Sum1/1  "int"
  Sum4/1 -> Anti-windup gain/1
  Ki/1 -> Sum5/2
  Anti-windup gain/1 -> Sum5/1
  Demux/2 -> Kd/1, Mux/2  "ev"
  Switch/1 -> Demux/1
  Mux1/1 -> Switch/1
  activate/1 -> Integrator1/2, Switch/2
  Constant/1 -> Switch/3
  Rate Limiter/1 -> u/1  "sat(u)"
  Compare To Constant1/1 -> AND/1
  Compare To Constant/1 -> AND/2
  Sum6/1 -> Integrator2/1, Kd1/1, Compare To Constant1/1
  Sum3/1 -> Switch1/1
  Integrator2/1 -> VelKi/1
  Kd1/1 -> Sum3/1
  VelKi/1 -> Sum3/2
  vMin/1 -> Sum6/1
  Switch1/1 -> Input Saturation/1  "u"
  error saturation/1 -> Kp/1, Ki/1
  Sum5/1 -> Integrator/1
  AND/1 -> Switch1/2, Integrator2/2
  [realInput] -> Sum4/2
  currentStates/1 -> Bus Selector/1
  Bus Selector/1 -> Headway error/1(xf)  "<X>"
  Bus Selector/2 -> Sum6/2, Headway error/2(vf), Sum/1  "<Xdot>"
  leaderStates/1 -> Bus Selector1/1
  Bus Selector1/1 -> Headway error/3(xl)  "<X>"
  Bus Selector/3 -> [realInput]  "<u>"
  lcFlag/1 -> Headway error/4(lcFlag)

== system gap_generation_platoon_alternative/p1/ACC ==
  note: Vehicle following
  note: Switch logic (veh foll to vel control)
  note: Velocity control
  note: If there's no leader or the leader
      | is too far away, use velocity control
  currentStates : Inport
  leaderStates : Inport  Port=2
  lcFlag : Inport  Port=3
  ACC outputs : Scope  NumInputPorts=3
  AND : Logic  IconShape=distinctive  AllPortsSameDT=off  OutDataTypeStr=boolean
  Anti-windup gain : Gain  Gain=sqrt(Ki/Kd)
  Bus Selector : BusSelector  OutputSignals=X,Xdot,u
  Bus Selector1 : BusSelector  OutputSignals=X,Xdot
  Compare To Constant : simulink/Logic and Bit Operations/Compare To Constant  relop=<  const=2*maxHeadwayError  OutDataTypeStr=boolean
  Compare To Constant1 : simulink/Logic and Bit Operations/Compare To Constant  relop=>  const=0  OutDataTypeStr=boolean
  Gain3 : Gain  Gain=velFilterGain
  Headway error : Subsystem
  Integrator : Integrator  ExternalReset=either
  Integrator1 : Integrator  InitialCondition=vx0
  Integrator2 : Integrator
  Kd : Gain  Gain=Kd
  Ki : Gain  Gain=Ki
  Kp : Gain  Gain=Kp
  Mux : Mux  Inputs=2
  Rate Limiter : RateLimiter  RisingSlewLimit=maxJerk  FallingSlewLimit=minJerk  SampleTimeMode=inherited
  Saturation : Saturate  UpperLimit=maxAcceleration  LowerLimit=minAcceleration
  Saturation1 : Saturate  UpperLimit=maxHeadwayError  LowerLimit=minHeadwayError
  Saturation2 : Saturate  UpperLimit=maxAcceleration  LowerLimit=minAcceleration
  Scope : Scope  NumInputPorts=3
  Sum : Sum  Inputs=-+|
  Sum1 : Sum  Inputs=+++
  Sum2 : Sum  Inputs=|+-
  Sum3 : Sum
  Sum4 : Sum  Inputs=+-
  Sum5 : Sum  Inputs=-+|
  Switch : Switch  Criteria=u2 > Threshold
  velKi : Gain  Gain=velKi
  velKp : Gain  Gain=velKp
  u : Outport
  errors : Outport  Port=2
  gap : Outport  Port=3
  wires:
  Headway error/1(eh) -> Mux/1, Compare To Constant/1, Saturation1/1
  Bus Selector/2 -> Headway error/2(vf), Sum/1  "<Xdot>"
  Kd/1 -> Scope/3, Sum1/3
  Kp/1 -> Scope/2, Sum1/2
  Gain3/1 -> Saturation/1
  Saturation/1 -> Integrator1/1
  Integrator1/1 -> Sum2/2, Sum/2
  Bus Selector1/2 -> Sum2/1  "<Xdot>"
  Sum2/1 -> Gain3/1
  Saturation1/1 -> Kp/1, Ki/1
  Headway error/2("gap ") -> gap/1
  Integrator2/1 -> velKi/1
  velKi/1 -> Sum3/2
  Switch/1 -> Sum4/1, Saturation2/1  "u"
  Sum1/1 -> Switch/1, ACC outputs/1
  Sum3/1 -> ACC outputs/3, Switch/3
  Sum/1 -> Mux/2, Kd/1, velKp/1, Integrator2/1
  Mux/1 -> errors/1
  Saturation2/1 -> Rate Limiter/1
  Sum4/1 -> Anti-windup gain/1
  Sum5/1 -> Integrator/1
  Rate Limiter/1 -> u/1  "sat(u)"
  velKp/1 -> Sum3/1
  Ki/1 -> Sum5/2
  Integrator/1 -> Sum1/1, Scope/1
  Anti-windup gain/1 -> Sum5/1
  AND/1 -> Integrator/2, Switch/2, ACC outputs/2
  Compare To Constant/1 -> AND/2
  Compare To Constant1/1 -> AND/1
  lcFlag/1 -> Headway error/4(lcFlag)
  currentStates/1 -> Bus Selector/1
  Bus Selector/1 -> Headway error/1(xf)  "<X>"
  leaderStates/1 -> Bus Selector1/1
  Bus Selector1/1 -> Compare To Constant1/1, Headway error/3(xl)  "<X>"
  Bus Selector/3 -> [realInput]  "<u>"
  [realInput] -> Sum4/2

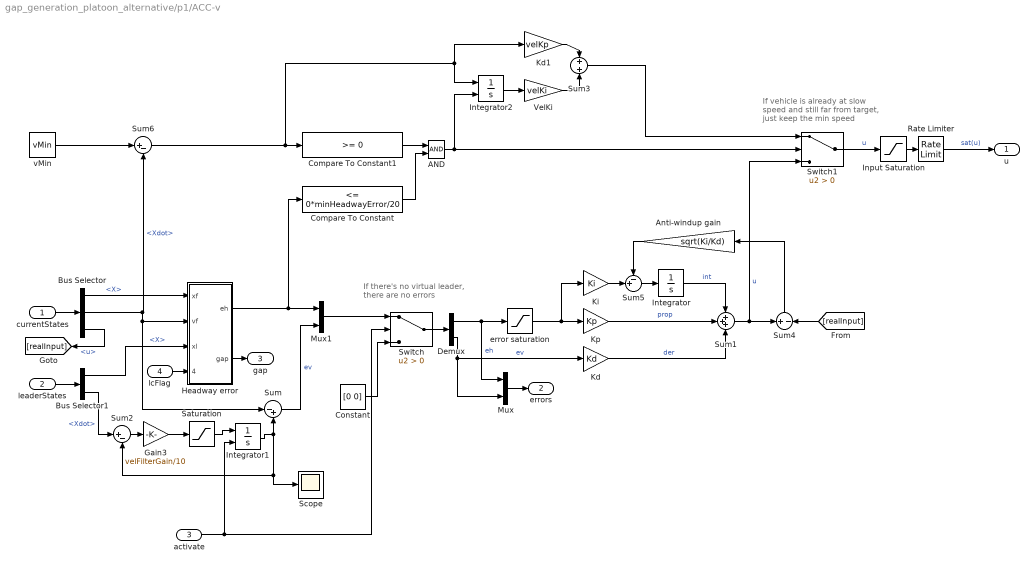
== system gap_generation_platoon_alternative/p1/ACC-v ==
  note: If vehicle is already at slow
      | speed and still far from target,
      | just keep the min speed
  note: If there's no virtual leader,
      | there are no errors
  currentStates : Inport
  leaderStates : Inport  Port=2
  activate : Inport  Port=3
  lcFlag : Inport  Port=4
  AND : Logic  IconShape=distinctive  AllPortsSameDT=off  OutDataTypeStr=boolean
  Anti-windup gain : Gain  Gain=sqrt(Ki/Kd)
  Bus Selector : BusSelector  OutputSignals=X,Xdot,u
  Bus Selector1 : BusSelector  OutputSignals=X,Xdot
  Compare To Constant : simulink/Logic and Bit Operations/Compare To Constant  relop=<=  const=0*minHeadwayError/20  OutDataTypeStr=boolean
  Compare To Constant1 : simulink/Logic and Bit Operations/Compare To Constant  relop=>=  const=0  OutDataTypeStr=boolean
  Constant : Constant  Value=[0 0]
  Demux : Demux  Outputs=2
  Gain3 : Gain  Gain=velFilterGain/10
  Headway error : Subsystem
  Input Saturation : Saturate  UpperLimit=maxAcceleration/2  LowerLimit=minAcceleration/4
  Integrator : Integrator
  Integrator1 : Integrator  ExternalReset=rising  InitialCondition=vx0
  Integrator2 : Integrator  ExternalReset=rising
  Kd : Gain  Gain=Kd
  Kd1 : Gain  Gain=velKp
  Ki : Gain  Gain=Ki
  Kp : Gain  Gain=Kp
  Mux : Mux  Inputs=2
  Mux1 : Mux  Inputs=2
  Rate Limiter : RateLimiter  RisingSlewLimit=maxJerk/2  FallingSlewLimit=minJerk/3  SampleTimeMode=inherited
  Saturation : Saturate  UpperLimit=maxAcceleration  LowerLimit=minAcceleration
  Scope : Scope
  Sum : Sum  Inputs=|-+
  Sum1 : Sum  Inputs=+++
  Sum2 : Sum  Inputs=|+-
  Sum3 : Sum
  Sum4 : Sum  Inputs=+-
  Sum5 : Sum  Inputs=-+|
  Sum6 : Sum  Inputs=|+-
  Switch : Switch  Criteria=u2 > Threshold
  Switch1 : Switch  Criteria=u2 > Threshold
  VelKi : Gain  Gain=velKi
  error saturation : Saturate  UpperLimit=maxHeadwayError  LowerLimit=minHeadwayError/10
  vMin : Constant  Value=vMin
  u : Outport
  errors : Outport  Port=2
  gap : Outport  Port=3
  wires:
  Headway error/1(eh) -> Compare To Constant/1, Mux1/1
  Kd/1 -> Sum1/3  "der"
  Kp/1 -> Sum1/2  "prop"
  Gain3/1 -> Saturation/1
  Saturation/1 -> Integrator1/1
  Integrator1/1 -> Scope/1, Sum2/2, Sum/2
  Bus Selector1/2 -> Sum2/1  "<Xdot>"
  Sum2/1 -> Gain3/1
  Demux/1 -> Mux/1, error saturation/1  "eh"
  Headway error/2("gap ") -> gap/1
  Sum1/1 -> Switch1/3, Sum4/1  "u"
  Sum/1 -> Mux1/2  "ev"
  Mux/1 -> errors/1
  Input Saturation/1 -> Rate Limiter/1
  Integrator/1 -> Sum1/1  "int"
  Sum4/1 -> Anti-windup gain/1
  Ki/1 -> Sum5/2
  Anti-windup gain/1 -> Sum5/1
  Demux/2 -> Kd/1, Mux/2  "ev"
  Switch/1 -> Demux/1
  Mux1/1 -> Switch/1
  activate/1 -> Integrator1/2, Switch/2
  Constant/1 -> Switch/3
  Rate Limiter/1 -> u/1  "sat(u)"
  Compare To Constant1/1 -> AND/1
  Compare To Constant/1 -> AND/2
  Sum6/1 -> Integrator2/1, Kd1/1, Compare To Constant1/1
  Sum3/1 -> Switch1/1
  Integrator2/1 -> VelKi/1
  Kd1/1 -> Sum3/1
  VelKi/1 -> Sum3/2
  vMin/1 -> Sum6/1
  Switch1/1 -> Input Saturation/1  "u"
  error saturation/1 -> Kp/1, Ki/1
  Sum5/1 -> Integrator/1
  AND/1 -> Switch1/2, Integrator2/2
  [realInput] -> Sum4/2
  currentStates/1 -> Bus Selector/1
  Bus Selector/1 -> Headway error/1(xf)  "<X>"
  Bus Selector/2 -> Sum6/2, Headway error/2(vf), Sum/1  "<Xdot>"
  leaderStates/1 -> Bus Selector1/1
  Bus Selector1/1 -> Headway error/3(xl)  "<X>"
  Bus Selector/3 -> [realInput]  "<u>"
  lcFlag/1 -> Headway error/4(lcFlag)

== system gap_generation_platoon_alternative/p1/Triggered Subsystem ==
  In1 : Inport
  Trigger : TriggerPort  VariantControl=Variant
  Out1 : Outport
  wires:
  In1/1 -> Out1/1

== system gap_generation_platoon_alternative/p2/ACC ==
  note: Vehicle following
  note: Switch logic (veh foll to vel control)
  note: Velocity control
  note: If there's no leader or the leader
      | is too far away, use velocity control
  currentStates : Inport
  leaderStates : Inport  Port=2
  lcFlag : Inport  Port=3
  ACC outputs : Scope  NumInputPorts=3
  AND : Logic  IconShape=distinctive  AllPortsSameDT=off  OutDataTypeStr=boolean
  Anti-windup gain : Gain  Gain=sqrt(Ki/Kd)
  Bus Selector : BusSelector  OutputSignals=X,Xdot,u
  Bus Selector1 : BusSelector  OutputSignals=X,Xdot
  Compare To Constant : simulink/Logic and Bit Operations/Compare To Constant  relop=<  const=2*maxHeadwayError  OutDataTypeStr=boolean
  Compare To Constant1 : simulink/Logic and Bit Operations/Compare To Constant  relop=>  const=0  OutDataTypeStr=boolean
  Gain3 : Gain  Gain=velFilterGain
  Headway error : Subsystem
  Integrator : Integrator  ExternalReset=either
  Integrator1 : Integrator  InitialCondition=vx0
  Integrator2 : Integrator
  Kd : Gain  Gain=Kd
  Ki : Gain  Gain=Ki
  Kp : Gain  Gain=Kp
  Mux : Mux  Inputs=2
  Rate Limiter : RateLimiter  RisingSlewLimit=maxJerk  FallingSlewLimit=minJerk  SampleTimeMode=inherited
  Saturation : Saturate  UpperLimit=maxAcceleration  LowerLimit=minAcceleration
  Saturation1 : Saturate  UpperLimit=maxHeadwayError  LowerLimit=minHeadwayError
  Saturation2 : Saturate  UpperLimit=maxAcceleration  LowerLimit=minAcceleration
  Scope : Scope  NumInputPorts=3
  Sum : Sum  Inputs=-+|
  Sum1 : Sum  Inputs=+++
  Sum2 : Sum  Inputs=|+-
  Sum3 : Sum
  Sum4 : Sum  Inputs=+-
  Sum5 : Sum  Inputs=-+|
  Switch : Switch  Criteria=u2 > Threshold
  velKi : Gain  Gain=velKi
  velKp : Gain  Gain=velKp
  u : Outport
  errors : Outport  Port=2
  gap : Outport  Port=3
  wires:
  Headway error/1(eh) -> Mux/1, Compare To Constant/1, Saturation1/1
  Bus Selector/2 -> Headway error/2(vf), Sum/1  "<Xdot>"
  Kd/1 -> Scope/3, Sum1/3
  Kp/1 -> Scope/2, Sum1/2
  Gain3/1 -> Saturation/1
  Saturation/1 -> Integrator1/1
  Integrator1/1 -> Sum2/2, Sum/2
  Bus Selector1/2 -> Sum2/1  "<Xdot>"
  Sum2/1 -> Gain3/1
  Saturation1/1 -> Kp/1, Ki/1
  Headway error/2("gap ") -> gap/1
  Integrator2/1 -> velKi/1
  velKi/1 -> Sum3/2
  Switch/1 -> Sum4/1, Saturation2/1  "u"
  Sum1/1 -> Switch/1, ACC outputs/1
  Sum3/1 -> ACC outputs/3, Switch/3
  Sum/1 -> Mux/2, Kd/1, velKp/1, Integrator2/1
  Mux/1 -> errors/1
  Saturation2/1 -> Rate Limiter/1
  Sum4/1 -> Anti-windup gain/1
  Sum5/1 -> Integrator/1
  Rate Limiter/1 -> u/1  "sat(u)"
  velKp/1 -> Sum3/1
  Ki/1 -> Sum5/2
  Integrator/1 -> Sum1/1, Scope/1
  Anti-windup gain/1 -> Sum5/1
  AND/1 -> Integrator/2, Switch/2, ACC outputs/2
  Compare To Constant/1 -> AND/2
  Compare To Constant1/1 -> AND/1
  lcFlag/1 -> Headway error/4(lcFlag)
  currentStates/1 -> Bus Selector/1
  Bus Selector/1 -> Headway error/1(xf)  "<X>"
  leaderStates/1 -> Bus Selector1/1
  Bus Selector1/1 -> Compare To Constant1/1, Headway error/3(xl)  "<X>"
  Bus Selector/3 -> [realInput]  "<u>"
  [realInput] -> Sum4/2

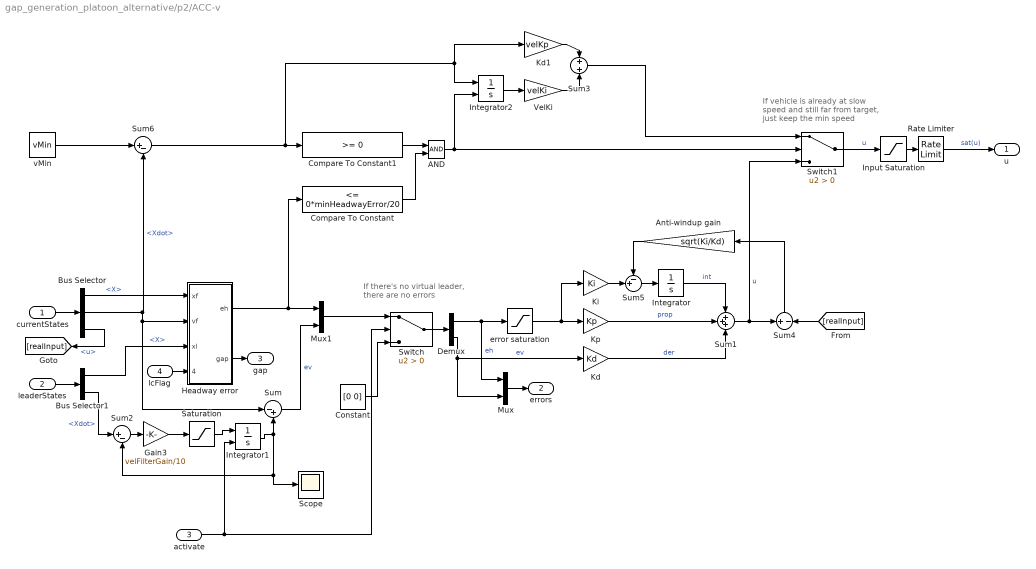
== system gap_generation_platoon_alternative/p2/ACC-v ==
  note: If vehicle is already at slow
      | speed and still far from target,
      | just keep the min speed
  note: If there's no virtual leader,
      | there are no errors
  currentStates : Inport
  leaderStates : Inport  Port=2
  activate : Inport  Port=3
  lcFlag : Inport  Port=4
  AND : Logic  IconShape=distinctive  AllPortsSameDT=off  OutDataTypeStr=boolean
  Anti-windup gain : Gain  Gain=sqrt(Ki/Kd)
  Bus Selector : BusSelector  OutputSignals=X,Xdot,u
  Bus Selector1 : BusSelector  OutputSignals=X,Xdot
  Compare To Constant : simulink/Logic and Bit Operations/Compare To Constant  relop=<=  const=0*minHeadwayError/20  OutDataTypeStr=boolean
  Compare To Constant1 : simulink/Logic and Bit Operations/Compare To Constant  relop=>=  const=0  OutDataTypeStr=boolean
  Constant : Constant  Value=[0 0]
  Demux : Demux  Outputs=2
  Gain3 : Gain  Gain=velFilterGain/10
  Headway error : Subsystem
  Input Saturation : Saturate  UpperLimit=maxAcceleration/2  LowerLimit=minAcceleration/4
  Integrator : Integrator
  Integrator1 : Integrator  ExternalReset=rising  InitialCondition=vx0
  Integrator2 : Integrator  ExternalReset=rising
  Kd : Gain  Gain=Kd
  Kd1 : Gain  Gain=velKp
  Ki : Gain  Gain=Ki
  Kp : Gain  Gain=Kp
  Mux : Mux  Inputs=2
  Mux1 : Mux  Inputs=2
  Rate Limiter : RateLimiter  RisingSlewLimit=maxJerk/2  FallingSlewLimit=minJerk/3  SampleTimeMode=inherited
  Saturation : Saturate  UpperLimit=maxAcceleration  LowerLimit=minAcceleration
  Scope : Scope
  Sum : Sum  Inputs=|-+
  Sum1 : Sum  Inputs=+++
  Sum2 : Sum  Inputs=|+-
  Sum3 : Sum
  Sum4 : Sum  Inputs=+-
  Sum5 : Sum  Inputs=-+|
  Sum6 : Sum  Inputs=|+-
  Switch : Switch  Criteria=u2 > Threshold
  Switch1 : Switch  Criteria=u2 > Threshold
  VelKi : Gain  Gain=velKi
  error saturation : Saturate  UpperLimit=maxHeadwayError  LowerLimit=minHeadwayError/10
  vMin : Constant  Value=vMin
  u : Outport
  errors : Outport  Port=2
  gap : Outport  Port=3
  wires:
  Headway error/1(eh) -> Compare To Constant/1, Mux1/1
  Kd/1 -> Sum1/3  "der"
  Kp/1 -> Sum1/2  "prop"
  Gain3/1 -> Saturation/1
  Saturation/1 -> Integrator1/1
  Integrator1/1 -> Scope/1, Sum2/2, Sum/2
  Bus Selector1/2 -> Sum2/1  "<Xdot>"
  Sum2/1 -> Gain3/1
  Demux/1 -> Mux/1, error saturation/1  "eh"
  Headway error/2("gap ") -> gap/1
  Sum1/1 -> Switch1/3, Sum4/1  "u"
  Sum/1 -> Mux1/2  "ev"
  Mux/1 -> errors/1
  Input Saturation/1 -> Rate Limiter/1
  Integrator/1 -> Sum1/1  "int"
  Sum4/1 -> Anti-windup gain/1
  Ki/1 -> Sum5/2
  Anti-windup gain/1 -> Sum5/1
  Demux/2 -> Kd/1, Mux/2  "ev"
  Switch/1 -> Demux/1
  Mux1/1 -> Switch/1
  activate/1 -> Integrator1/2, Switch/2
  Constant/1 -> Switch/3
  Rate Limiter/1 -> u/1  "sat(u)"
  Compare To Constant1/1 -> AND/1
  Compare To Constant/1 -> AND/2
  Sum6/1 -> Integrator2/1, Kd1/1, Compare To Constant1/1
  Sum3/1 -> Switch1/1
  Integrator2/1 -> VelKi/1
  Kd1/1 -> Sum3/1
  VelKi/1 -> Sum3/2
  vMin/1 -> Sum6/1
  Switch1/1 -> Input Saturation/1  "u"
  error saturation/1 -> Kp/1, Ki/1
  Sum5/1 -> Integrator/1
  AND/1 -> Switch1/2, Integrator2/2
  [realInput] -> Sum4/2
  currentStates/1 -> Bus Selector/1
  Bus Selector/1 -> Headway error/1(xf)  "<X>"
  Bus Selector/2 -> Sum6/2, Headway error/2(vf), Sum/1  "<Xdot>"
  leaderStates/1 -> Bus Selector1/1
  Bus Selector1/1 -> Headway error/3(xl)  "<X>"
  Bus Selector/3 -> [realInput]  "<u>"
  lcFlag/1 -> Headway error/4(lcFlag)

== system gap_generation_platoon_alternative/p2/Triggered Subsystem ==
  In1 : Inport
  Trigger : TriggerPort  VariantControl=Variant
  Out1 : Outport
  wires:
  In1/1 -> Out1/1

== system gap_generation_platoon_alternative/p3/ACC ==
  note: Vehicle following
  note: Switch logic (veh foll to vel control)
  note: Velocity control
  note: If there's no leader or the leader
      | is too far away, use velocity control
  currentStates : Inport
  leaderStates : Inport  Port=2
  lcFlag : Inport  Port=3
  ACC outputs : Scope  NumInputPorts=3
  AND : Logic  IconShape=distinctive  AllPortsSameDT=off  OutDataTypeStr=boolean
  Anti-windup gain : Gain  Gain=sqrt(Ki/Kd)
  Bus Selector : BusSelector  OutputSignals=X,Xdot,u
  Bus Selector1 : BusSelector  OutputSignals=X,Xdot
  Compare To Constant : simulink/Logic and Bit Operations/Compare To Constant  relop=<  const=2*maxHeadwayError  OutDataTypeStr=boolean
  Compare To Constant1 : simulink/Logic and Bit Operations/Compare To Constant  relop=>  const=0  OutDataTypeStr=boolean
  Gain3 : Gain  Gain=velFilterGain
  Headway error : Subsystem
  Integrator : Integrator  ExternalReset=either
  Integrator1 : Integrator  InitialCondition=vx0
  Integrator2 : Integrator
  Kd : Gain  Gain=Kd
  Ki : Gain  Gain=Ki
  Kp : Gain  Gain=Kp
  Mux : Mux  Inputs=2
  Rate Limiter : RateLimiter  RisingSlewLimit=maxJerk  FallingSlewLimit=minJerk  SampleTimeMode=inherited
  Saturation : Saturate  UpperLimit=maxAcceleration  LowerLimit=minAcceleration
  Saturation1 : Saturate  UpperLimit=maxHeadwayError  LowerLimit=minHeadwayError
  Saturation2 : Saturate  UpperLimit=maxAcceleration  LowerLimit=minAcceleration
  Scope : Scope  NumInputPorts=3
  Sum : Sum  Inputs=-+|
  Sum1 : Sum  Inputs=+++
  Sum2 : Sum  Inputs=|+-
  Sum3 : Sum
  Sum4 : Sum  Inputs=+-
  Sum5 : Sum  Inputs=-+|
  Switch : Switch  Criteria=u2 > Threshold
  velKi : Gain  Gain=velKi
  velKp : Gain  Gain=velKp
  u : Outport
  errors : Outport  Port=2
  gap : Outport  Port=3
  wires:
  Headway error/1(eh) -> Mux/1, Compare To Constant/1, Saturation1/1
  Bus Selector/2 -> Headway error/2(vf), Sum/1  "<Xdot>"
  Kd/1 -> Scope/3, Sum1/3
  Kp/1 -> Scope/2, Sum1/2
  Gain3/1 -> Saturation/1
  Saturation/1 -> Integrator1/1
  Integrator1/1 -> Sum2/2, Sum/2
  Bus Selector1/2 -> Sum2/1  "<Xdot>"
  Sum2/1 -> Gain3/1
  Saturation1/1 -> Kp/1, Ki/1
  Headway error/2("gap ") -> gap/1
  Integrator2/1 -> velKi/1
  velKi/1 -> Sum3/2
  Switch/1 -> Sum4/1, Saturation2/1  "u"
  Sum1/1 -> Switch/1, ACC outputs/1
  Sum3/1 -> ACC outputs/3, Switch/3
  Sum/1 -> Mux/2, Kd/1, velKp/1, Integrator2/1
  Mux/1 -> errors/1
  Saturation2/1 -> Rate Limiter/1
  Sum4/1 -> Anti-windup gain/1
  Sum5/1 -> Integrator/1
  Rate Limiter/1 -> u/1  "sat(u)"
  velKp/1 -> Sum3/1
  Ki/1 -> Sum5/2
  Integrator/1 -> Sum1/1, Scope/1
  Anti-windup gain/1 -> Sum5/1
  AND/1 -> Integrator/2, Switch/2, ACC outputs/2
  Compare To Constant/1 -> AND/2
  Compare To Constant1/1 -> AND/1
  lcFlag/1 -> Headway error/4(lcFlag)
  currentStates/1 -> Bus Selector/1
  Bus Selector/1 -> Headway error/1(xf)  "<X>"
  leaderStates/1 -> Bus Selector1/1
  Bus Selector1/1 -> Compare To Constant1/1, Headway error/3(xl)  "<X>"
  Bus Selector/3 -> [realInput]  "<u>"
  [realInput] -> Sum4/2

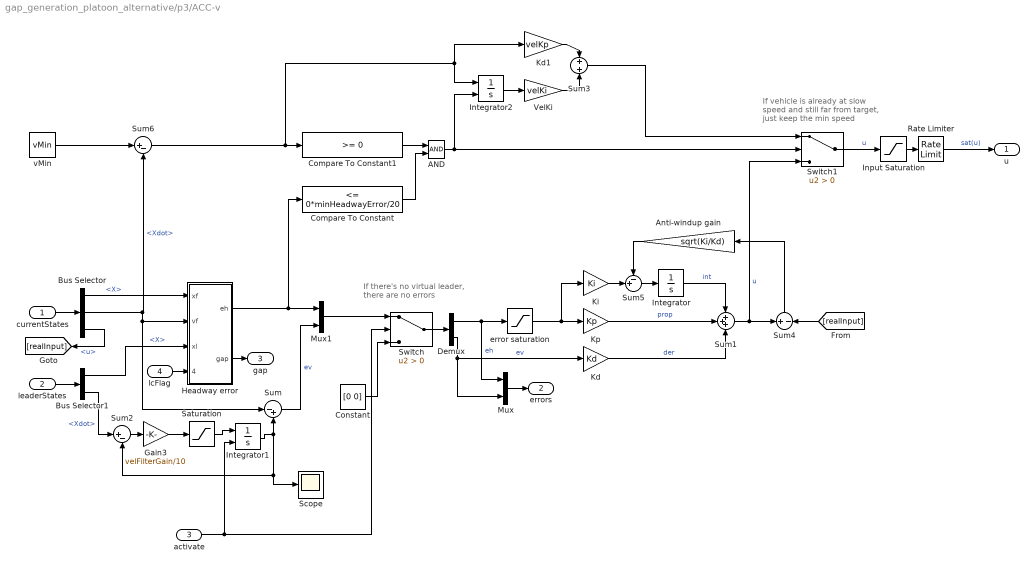
== system gap_generation_platoon_alternative/p3/ACC-v ==
  note: If vehicle is already at slow
      | speed and still far from target,
      | just keep the min speed
  note: If there's no virtual leader,
      | there are no errors
  currentStates : Inport
  leaderStates : Inport  Port=2
  activate : Inport  Port=3
  lcFlag : Inport  Port=4
  AND : Logic  IconShape=distinctive  AllPortsSameDT=off  OutDataTypeStr=boolean
  Anti-windup gain : Gain  Gain=sqrt(Ki/Kd)
  Bus Selector : BusSelector  OutputSignals=X,Xdot,u
  Bus Selector1 : BusSelector  OutputSignals=X,Xdot
  Compare To Constant : simulink/Logic and Bit Operations/Compare To Constant  relop=<=  const=0*minHeadwayError/20  OutDataTypeStr=boolean
  Compare To Constant1 : simulink/Logic and Bit Operations/Compare To Constant  relop=>=  const=0  OutDataTypeStr=boolean
  Constant : Constant  Value=[0 0]
  Demux : Demux  Outputs=2
  Gain3 : Gain  Gain=velFilterGain/10
  Headway error : Subsystem
  Input Saturation : Saturate  UpperLimit=maxAcceleration/2  LowerLimit=minAcceleration/4
  Integrator : Integrator
  Integrator1 : Integrator  ExternalReset=rising  InitialCondition=vx0
  Integrator2 : Integrator  ExternalReset=rising
  Kd : Gain  Gain=Kd
  Kd1 : Gain  Gain=velKp
  Ki : Gain  Gain=Ki
  Kp : Gain  Gain=Kp
  Mux : Mux  Inputs=2
  Mux1 : Mux  Inputs=2
  Rate Limiter : RateLimiter  RisingSlewLimit=maxJerk/2  FallingSlewLimit=minJerk/3  SampleTimeMode=inherited
  Saturation : Saturate  UpperLimit=maxAcceleration  LowerLimit=minAcceleration
  Scope : Scope
  Sum : Sum  Inputs=|-+
  Sum1 : Sum  Inputs=+++
  Sum2 : Sum  Inputs=|+-
  Sum3 : Sum
  Sum4 : Sum  Inputs=+-
  Sum5 : Sum  Inputs=-+|
  Sum6 : Sum  Inputs=|+-
  Switch : Switch  Criteria=u2 > Threshold
  Switch1 : Switch  Criteria=u2 > Threshold
  VelKi : Gain  Gain=velKi
  error saturation : Saturate  UpperLimit=maxHeadwayError  LowerLimit=minHeadwayError/10
  vMin : Constant  Value=vMin
  u : Outport
  errors : Outport  Port=2
  gap : Outport  Port=3
  wires:
  Headway error/1(eh) -> Compare To Constant/1, Mux1/1
  Kd/1 -> Sum1/3  "der"
  Kp/1 -> Sum1/2  "prop"
  Gain3/1 -> Saturation/1
  Saturation/1 -> Integrator1/1
  Integrator1/1 -> Scope/1, Sum2/2, Sum/2
  Bus Selector1/2 -> Sum2/1  "<Xdot>"
  Sum2/1 -> Gain3/1
  Demux/1 -> Mux/1, error saturation/1  "eh"
  Headway error/2("gap ") -> gap/1
  Sum1/1 -> Switch1/3, Sum4/1  "u"
  Sum/1 -> Mux1/2  "ev"
  Mux/1 -> errors/1
  Input Saturation/1 -> Rate Limiter/1
  Integrator/1 -> Sum1/1  "int"
  Sum4/1 -> Anti-windup gain/1
  Ki/1 -> Sum5/2
  Anti-windup gain/1 -> Sum5/1
  Demux/2 -> Kd/1, Mux/2  "ev"
  Switch/1 -> Demux/1
  Mux1/1 -> Switch/1
  activate/1 -> Integrator1/2, Switch/2
  Constant/1 -> Switch/3
  Rate Limiter/1 -> u/1  "sat(u)"
  Compare To Constant1/1 -> AND/1
  Compare To Constant/1 -> AND/2
  Sum6/1 -> Integrator2/1, Kd1/1, Compare To Constant1/1
  Sum3/1 -> Switch1/1
  Integrator2/1 -> VelKi/1
  Kd1/1 -> Sum3/1
  VelKi/1 -> Sum3/2
  vMin/1 -> Sum6/1
  Switch1/1 -> Input Saturation/1  "u"
  error saturation/1 -> Kp/1, Ki/1
  Sum5/1 -> Integrator/1
  AND/1 -> Switch1/2, Integrator2/2
  [realInput] -> Sum4/2
  currentStates/1 -> Bus Selector/1
  Bus Selector/1 -> Headway error/1(xf)  "<X>"
  Bus Selector/2 -> Sum6/2, Headway error/2(vf), Sum/1  "<Xdot>"
  leaderStates/1 -> Bus Selector1/1
  Bus Selector1/1 -> Headway error/3(xl)  "<X>"
  Bus Selector/3 -> [realInput]  "<u>"
  lcFlag/1 -> Headway error/4(lcFlag)
